simulink model "l1_lbw1_ver100"  (Simulink 7.9)
settings: Solver=FixedStepDiscrete  SolverMode=SingleTasking  StartTime=0.0  StopTime=16484  RelTol=1e-3
undefined symbols (not defined in the file): sfp
libraries: xbsIndex_r4 x1286, casper_library_downconverter x92, dspsigops x32, xps_library x22, casper_library_misc x18, casper_library_flow_control x4
(part 1 of 10)
settings Model: Creator=jayanth  LastModifiedBy=mwagner
settings DebuggingCC: FcnCallInpInsideContextMsg=Use local settings
settings GRTTargetCC: CombineOutputUpdateFcns=off  GRTInterface=on

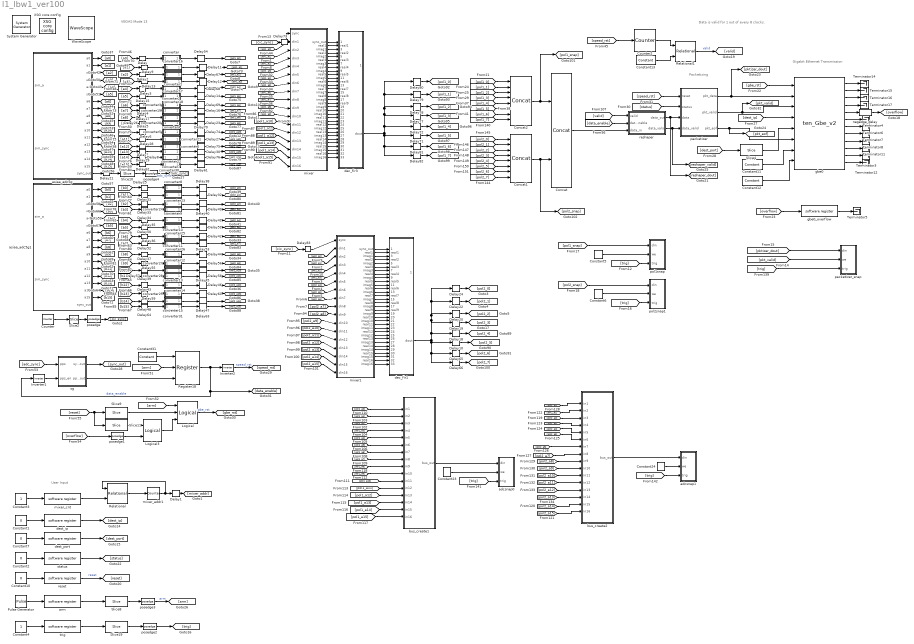
== system l1_lbw1_ver100 ==
  note: Gigabit Ethernet Transmission
  note: Packetizing
  note: Data is valid for 1 out of every 8 clocks.
  note: VEGAS Mode 13
  note: User Input
  " System Generator" : xbsIndex_r4/ System Generator  Tag=genX  xilinxfamily=virtex6  part=xc6vsx475t  speed=-1  package=ff1759  synthesis_tool=XST  clock_wrapper=Clock Enables  directory=./v13_16r128dr_ver110/sysgen  proj_type=Project Navigator  Synth_file=XST Defaults  Impl_file=ISE Defaults  testbench=off  simulink_period=1  sysclk_period=6.6667  dcm_input_clock_period=100  incr_netlist=off  trim_vbits=Everywhere in SubSystem  dbl_ovrd=According to Block Masks  core_generation=According to Block Masks  run_coregen=off  deprecated_control=off  eval_field=0  block_type=sysgen
  Concat : xbsIndex_r4/Concat  num_inputs=2  dbl_ovrd=off  block_type=concat
  Concat1 : xbsIndex_r4/Concat  num_inputs=8  dbl_ovrd=off  block_type=concat
  Concat2 : xbsIndex_r4/Concat  num_inputs=8  dbl_ovrd=off  block_type=concat
  Constant{1..2,7,10} (4 alike) : Constant  Value=0
  Constant11 : xbsIndex_r4/Constant  const=1  gui_display_data_type=Boolean  arith_type=Boolean  n_bits=16  bin_pt=14  preci_type=Single  exp_width=8  frac_width=24  explicit_period=on  period=1  equ=P=C  opselect=C  inp2=PCIN>>17  opr=+  inp1=P  carry=CIN  dbl_ovrd=off  block_type=constant
  Constant12 : xbsIndex_r4/Constant  const=0  gui_display_data_type=Boolean  arith_type=Boolean  n_bits=16  bin_pt=14  preci_type=Single  exp_width=8  frac_width=24  explicit_period=on  period=1  equ=P=C  opselect=C  inp2=PCIN>>17  opr=+  inp1=P  carry=CIN  dbl_ovrd=off  block_type=constant
  Constant13 : xbsIndex_r4/Constant  const=7  gui_display_data_type=Fixed-point  arith_type=Unsigned  n_bits=3  bin_pt=0  preci_type=Single  exp_width=8  frac_width=24  explicit_period=on  period=1  equ=P=C  opselect=C  inp2=PCIN>>17  opr=+  inp1=P  carry=CIN  dbl_ovrd=off  block_type=constant
  Constant{5..6,23..24} (4 alike) : xbsIndex_r4/Constant  const=1  gui_display_data_type=Boolean  arith_type=Boolean  n_bits=32  bin_pt=0  preci_type=Single  exp_width=8  frac_width=24  explicit_period=on  period=1  equ=P=C  opselect=C  inp2=PCIN>>17  opr=+  inp1=P  carry=CIN  dbl_ovrd=off  block_type=constant
      settings: block_version=11.4
  Constant3 : Constant
  Constant31 : xbsIndex_r4/Constant  const=1  gui_display_data_type=Fixed-point  arith_type=Boolean  n_bits=16  bin_pt=0  preci_type=Single  exp_width=8  frac_width=24  explicit_period=on  period=1  equ=P=C  opselect=C  inp2=PCIN>>17  opr=+  inp1=P  carry=CIN  dbl_ovrd=off  block_type=constant
      settings: block_version=11.4
  Constant4 : Constant
  Counter : xbsIndex_r4/Counter  cnt_type=Free Running  cnt_to=Inf  operation=Up  start_count=0  cnt_by_val=1  arith_type=Unsigned  n_bits=16  bin_pt=0  load_pin=off  rst=off  en=off  explicit_period=on  period=1  dbl_ovrd=off  use_behavioral_HDL=off  implementation=Fabric  block_type=counter
  Counter2 : xbsIndex_r4/Counter  cnt_type=Free Running  cnt_to=Inf  operation=Up  start_count=5  cnt_by_val=1  arith_type=Unsigned  n_bits=3  bin_pt=0  load_pin=off  rst=on  en=off  explicit_period=on  period=1  dbl_ovrd=off  use_behavioral_HDL=off  implementation=Fabric  block_type=counter
      settings: block_version=11.4
  Delay{,2..9,13,15,17,21,25..26,28..29,31,33..37,39,43,48,50,52,55,57,59,62,64} (33 alike) : xbsIndex_r4/Delay  rst=off  infoeditControl=Selection of Reset will increase slice count due to use of real FFs and instead of SRLs  en=off  latency=3  dbl_ovrd=off  reg_retiming=off  block_type=delay
  Delay1 : xbsIndex_r4/Delay  rst=off  infoeditControl=Selection of Reset will increase slice count due to use of real FFs and instead of SRLs  en=off  latency=2  dbl_ovrd=off  reg_retiming=on  block_type=delay
      settings: block_version=11.4
  Delay10 : xbsIndex_r4/Delay  rst=off  infoeditControl=Selection of Reset will increase slice count due to use of real FFs and instead of SRLs  en=off  latency=6  dbl_ovrd=off  reg_retiming=on  block_type=delay
      settings: block_version=11.4
  Delay{11..12,14,16,20,23,27,30,32,38,40..42,44..47,49,51,53..54,56,58,60..61,63,67..70,74..76,78} (34 alike) : xbsIndex_r4/Delay  rst=off  infoeditControl=Selection of Reset will increase slice count due to use of real FFs and instead of SRLs  en=off  latency=3  dbl_ovrd=off  reg_retiming=on  block_type=delay
      settings: block_version=11.4
  Delay{18,72..73,83} (4 alike) : xbsIndex_r4/Delay  rst=off  infoeditControl=Selection of Reset will increase slice count due to use of real FFs and instead of SRLs  en=off  latency=5  dbl_ovrd=off  reg_retiming=on  block_type=delay
      settings: block_version=11.4
  Delay19 : xbsIndex_r4/Delay  rst=off  infoeditControl=Selection of Reset will increase slice count due to use of real FFs and instead of SRLs  en=off  latency=4  dbl_ovrd=off  reg_retiming=on  block_type=delay
      settings: block_version=11.4
  Delay22 : xbsIndex_r4/Delay  rst=off  infoeditControl=Selection of Reset will increase slice count due to use of real FFs and instead of SRLs  en=off  latency=2  dbl_ovrd=off  reg_retiming=on  block_type=delay
      settings: block_version=11.4
  Delay24 : xbsIndex_r4/Delay  rst=off  infoeditControl=Selection of Reset will increase slice count due to use of real FFs and instead of SRLs  en=off  latency=1  dbl_ovrd=off  reg_retiming=on  block_type=delay
      settings: block_version=11.4
  Delay65 : xbsIndex_r4/Delay  rst=off  infoeditControl=Selection of Reset will increase slice count due to use of real FFs and instead of SRLs  en=off  latency=7  dbl_ovrd=off  reg_retiming=on  block_type=delay
      settings: block_version=11.4
  Delay66 : xbsIndex_r4/Delay  rst=off  infoeditControl=Selection of Reset will increase slice count due to use of real FFs and instead of SRLs  en=off  latency=8  dbl_ovrd=off  reg_retiming=on  block_type=delay
      settings: block_version=11.4
  Delay71 : xbsIndex_r4/Delay  rst=off  infoeditControl=Selection of Reset will increase slice count due to use of real FFs and instead of SRLs  en=off  latency=6  dbl_ovrd=off  reg_retiming=on  block_type=delay
      settings: block_version=11.4
  Delay77 : xbsIndex_r4/Delay  rst=off  infoeditControl=Selection of Reset will increase slice count due to use of real FFs and instead of SRLs  en=off  latency=4  dbl_ovrd=off  reg_retiming=on  block_type=delay
      settings: block_version=11.4
  Delay79 : xbsIndex_r4/Delay  rst=off  infoeditControl=Selection of Reset will increase slice count due to use of real FFs and instead of SRLs  en=off  latency=2  dbl_ovrd=off  reg_retiming=on  block_type=delay
      settings: block_version=11.4
  Delay80 : xbsIndex_r4/Delay  rst=off  infoeditControl=Selection of Reset will increase slice count due to use of real FFs and instead of SRLs  en=off  latency=1  dbl_ovrd=off  reg_retiming=on  block_type=delay
      settings: block_version=11.4
  Delay81 : xbsIndex_r4/Delay  rst=off  infoeditControl=Selection of Reset will increase slice count due to use of real FFs and instead of SRLs  en=off  latency=7  dbl_ovrd=off  reg_retiming=on  block_type=delay
      settings: block_version=11.4
  Delay82 : xbsIndex_r4/Delay  rst=off  infoeditControl=Selection of Reset will increase slice count due to use of real FFs and instead of SRLs  en=off  latency=8  dbl_ovrd=off  reg_retiming=on  block_type=delay
      settings: block_version=11.4
  Inverter1 : xbsIndex_r4/Inverter  en=off  latency=0  dbl_ovrd=off  block_type=inv
      settings: block_version=11.4
  Inverter2 : xbsIndex_r4/Inverter  en=off  latency=0  dbl_ovrd=off  block_type=inv
      settings: block_version=11.4
  Logical : xbsIndex_r4/Logical  logical_function=OR  inputs=3  en=off  latency=0  precision=Full  arith_type=Unsigned  n_bits=16  bin_pt=0  align_bp=on  dbl_ovrd=off  block_type=logical
  Logical3 : xbsIndex_r4/Logical  logical_function=AND  inputs=2  en=off  latency=0  precision=Full  arith_type=Unsigned  n_bits=8  bin_pt=2  align_bp=on  dbl_ovrd=off  block_type=logical
      settings: xl_area=[0, 0, 0, 0, 0, 0, 0]
  Pulse Generator : DiscretePulseGenerator  Period=10000  PhaseDelay=100
  Register18 : xbsIndex_r4/Register  init=0  rst=on  en=on  dbl_ovrd=off  block_type=register
      settings: block_version=11.4
  Relational : xbsIndex_r4/Relational  mode=a=b  en=off  latency=1  dbl_ovrd=off  block_type=relational
  Relational1 : xbsIndex_r4/Relational  mode=a=b  en=off  latency=0  dbl_ovrd=off  block_type=relational
  Slice{8..10,19} (4 alike) : xbsIndex_r4/Slice  nbits=1  boolean_output=on  mode=Lower Bit Location + Width  bit1=0  base1=MSB of Input  bit0=0  base0=LSB of Input  dbl_ovrd=off  block_type=slice
  Slice11 : xbsIndex_r4/Slice  nbits=1  boolean_output=on  mode=Lower Bit Location + Width  bit1=0  base1=MSB of Input  bit0=1  base0=LSB of Input  dbl_ovrd=off  block_type=slice
      settings: block_version=10.1.3
  Slice2 : xbsIndex_r4/Slice  nbits=1  boolean_output=on  mode=Upper Bit Location + Width  bit1=0  base1=MSB of Input  bit0=0  base0=LSB of Input  dbl_ovrd=off  block_type=slice
  Slice4 : xbsIndex_r4/Slice  nbits=16  boolean_output=off  mode=Lower Bit Location + Width  bit1=0  base1=MSB of Input  bit0=0  base0=LSB of Input  dbl_ovrd=off  block_type=slice
  Terminator{3..8,11..12,14..17} (12 alike) : Terminator
  WaveScope : xbsIndex_r4/WaveScope  block_type=wavescope
  XSG core config : xps_library/XSG core config  Tag=xps:xsg  hw_sys=ROACH2:sx475t  clk_src=adc0_clk  ROACH_clk_src=adc0_clk  ROACH2_clk_src=adc0_clk  clk_rate=150  sample_period=1  synthesis_tool=XST
  adcsnap0 : Subsystem  AncestorBlock=casper_library_scopes/snapshot  mask(snapshot){storage=bram, dram_dimm=1, dram_clock=200, nsamples=12, data_width=128, offset=off, circap=off, value=off, use_dsp48=on}
      mask prompts: storage "Storage medium"; dram_dimm "DRAM dimm"; dram_clock "DRAM clock rate"; nsamples "Number of Samples (2^?)"; data_width "Data width"; offset "Start delay support"; circap "Circular capture support"; value "Extra value capture support"; use_dsp48 "Use DSP48s to implement counters"
      mask help:
      | Standard snap block, but with the following optional extras;
      |  1) Optionally delay the fabric trigger by a user-specified number of valids.
      |  2) Capture continuously after a trigger until a stop pulse is received. Data is captured into BRAM continuously, with old data being overwritten until a stop command is received. Then stop capturing when memory is filled. This enables you to get some data before and some data after the stop pulse. Use the 'tr_en_cnt' register to determine where you are in your vector. 'Addr' register's MSb now indicates 'busy capturing'.
      |  3) Optionally capture a value on an input port to a register at the same time as the first data sample.
      |  4) Implement counters using DSP48Es to save resources.
      mask init:
      | snapshot_init(gcb, ...
      |     'storage', storage, ...
      |     'dram_dimm', dram_dimm, ...
      |     'dram_clock', dram_clock, ...
      |     'nsamples', nsamples, ...
      |     'data_width', data_width, ...
      |     'offset', offset, ...
      |     'circap', circap, ...
      |     'value', value, ...
      |     'use_dsp48', use_dsp48);
      mask StyleString: popup(bram|dram),popup(1|2|3|4),popup(200|250|266|300|333),edit,popup(8|16|32|64|128),checkbox,checkbox,checkbox,checkbox
      mask CallbackString: snapshot_callback();||||||||
  adcsnap1 : Subsystem  AncestorBlock=casper_library_scopes/snapshot  mask(snapshot){storage=bram, dram_dimm=1, dram_clock=200, nsamples=12, data_width=128, offset=off, circap=off, value=off, use_dsp48=on}
      mask prompts: storage "Storage medium"; dram_dimm "DRAM dimm"; dram_clock "DRAM clock rate"; nsamples "Number of Samples (2^?)"; data_width "Data width"; offset "Start delay support"; circap "Circular capture support"; value "Extra value capture support"; use_dsp48 "Use DSP48s to implement counters"
      mask help:
      | Standard snap block, but with the following optional extras;
      |  1) Optionally delay the fabric trigger by a user-specified number of valids.
      |  2) Capture continuously after a trigger until a stop pulse is received. Data is captured into BRAM continuously, with old data being overwritten until a stop command is received. Then stop capturing when memory is filled. This enables you to get some data before and some data after the stop pulse. Use the 'tr_en_cnt' register to determine where you are in your vector. 'Addr' register's MSb now indicates 'busy capturing'.
      |  3) Optionally capture a value on an input port to a register at the same time as the first data sample.
      |  4) Implement counters using DSP48Es to save resources.
      mask init: same as l1_lbw1_ver100/adcsnap0
      mask StyleString: popup(bram|dram),popup(1|2|3|4),popup(200|250|266|300|333),edit,popup(8|16|32|64|128),checkbox,checkbox,checkbox,checkbox
      mask CallbackString: snapshot_callback();||||||||
  arm : xps_library/software register  Tag=xps:sw_reg  io_dir=From Processor  arith_type=Unsigned  bitwidth=32  bin_pt=0  sample_period=1  gw_name=h16k_hbw_ver100_arm_user_data_out
      link override convert: arith_type=Unsigned  n_bits=32  bin_pt=0
      link override newmode13_arm_user_data_out: arith_type=Unsigned  n_bits=32  bin_pt=0  period=1
      link override r_spec_2048_r102_cnt_rst_user_data_out: arith_type=Unsigned  n_bits=32  bin_pt=0  period=1
      link override r_spec_2048_r102_nosim_cnt_rst_user_data_out: arith_type=Unsigned  n_bits=32  bin_pt=0  period=1
      link override r_spec_2048_r103_cnt_rst_user_data_out: arith_type=Unsigned  n_bits=32  bin_pt=0  period=1
      link override roach_spec_no10gbe_sync_cnt_rst_user_data_out: arith_type=Unsigned  n_bits=32  bin_pt=0  period=1
      link override roach_spec_rst_cnt_user_data_out: arith_type=Unsigned  n_bits=32  bin_pt=0  period=1
      link override roach_spec_rst_sync_cnt_user_data_out: arith_type=Unsigned  n_bits=32  bin_pt=0  period=1
  asiaa_adc5g : Subsystem  Tag=xps:adc5g  AncestorBlock=xps_library/ADCs/asiaa_adc5g  mask(adc5g){input_mode=One-channel -- A, adc_brd=ZDOK 0, demux=1:1, adc_bit_width=8, adc_clk_rate=800, using_ctrl=on, test_ramp=off}
      mask prompts: input_mode "Input mode:"; adc_brd "ADC Board"; demux "Internal demux"; adc_bit_width "ADC Resolution (bits):"; adc_clk_rate "ADC Clock Rate (MHz):"; using_ctrl "use control"; test_ramp "start in test ramp mode"
      mask help:
      | Interface for the ASIAA 5 GSps ADC. Supports interleaving all four
      | cores using either input A or C, or interleaving two-cores each for
      | A and C. The hardware itself comes in two versions:
      |
      | DMUX 1:2 -- 4-bit samples, 4 parallel streams
      | DMUX 1:1 -- 8-bit samples, 2 parallel streams
      |
      | In either configuration this block will output 8 parallel streams
      | but the underlying interface, and the bitwidth of the samples,
      | will be different.
      mask init:
      | adc5g_init(gcb,...
      |     'input_mode', input_mode,...
      |     'demux', demux,...
      |     'adc_clk_rate', adc_clk_rate,...
      |     'adc_bit_width', adc_bit_width,...
      |     'adc_brd', adc_brd,...
      |     'using_ctrl', using_ctrl,...
      |     'test_ramp', test_ramp);
      mask StyleString: popup(One-channel -- A|One-channel -- C|Two-channel -- A&C),popup(ZDOK 0|ZDOK 1),popup(1:1|1:2),edit,edit,checkbox,checkbox
      mask CallbackString:
      | ||demux = get_param(gcb,'demux');
      | if(strcmp(demux,'1:1')),
      |     set_param(gcb, 'adc_bit_width', '8')
      | elseif(strcmp(demux, '1:2')),
      |     set_param(gcb, 'adc_bit_width', '4');
      | else
      | end||||
  asiaa_adc5g1 : Subsystem  Tag=xps:adc5g  AncestorBlock=xps_library/ADCs/asiaa_adc5g  mask(adc5g){input_mode=One-channel -- A, adc_brd=ZDOK 1, demux=1:1, adc_bit_width=8, adc_clk_rate=800, using_ctrl=on, test_ramp=off}
      mask prompts: input_mode "Input mode:"; adc_brd "ADC Board"; demux "Internal demux"; adc_bit_width "ADC Resolution (bits):"; adc_clk_rate "ADC Clock Rate (MHz):"; using_ctrl "use control"; test_ramp "start in test ramp mode"
      mask help:
      | Interface for the ASIAA 5 GSps ADC. Supports interleaving all four
      | cores using either input A or C, or interleaving two-cores each for
      | A and C. The hardware itself comes in two versions:
      |
      | DMUX 1:2 -- 4-bit samples, 4 parallel streams
      | DMUX 1:1 -- 8-bit samples, 2 parallel streams
      |
      | In either configuration this block will output 8 parallel streams
      | but the underlying interface, and the bitwidth of the samples,
      | will be different.
      mask init: same as l1_lbw1_ver100/asiaa_adc5g
      mask StyleString: popup(One-channel -- A|One-channel -- C|Two-channel -- A&C),popup(ZDOK 0|ZDOK 1),popup(1:1|1:2),edit,edit,checkbox,checkbox
      mask CallbackString:
      | ||demux = get_param(gcb,'demux');
      | if(strcmp(demux,'1:1')),
      |     set_param(gcb, 'adc_bit_width', '8')
      | elseif(strcmp(demux, '1:2')),
      |     set_param(gcb, 'adc_bit_width', '4');
      | else
      | end||||
  bus_create1 : Subsystem  AncestorBlock=casper_library_flow_control/bus_create  mask(bus_create){inputNum=16}
      mask prompts: inputNum "Number of inputs:"
      mask init:
      | bus_create_init(gcb,...
      |     'inputNum', inputNum);
  bus_create2 : Subsystem  AncestorBlock=casper_library_flow_control/bus_create  mask(bus_create){inputNum=16}
      mask prompts: inputNum "Number of inputs:"
      mask init:
      | bus_create_init(gcb,...
      |     'inputNum', inputNum);
  converter : Subsystem
  converter1 : Subsystem
  converter10 : Subsystem
  converter11 : Subsystem
  converter12 : Subsystem
  converter13 : Subsystem
  converter14 : Subsystem
  converter15 : Subsystem
  converter16 : Subsystem
  converter17 : Subsystem
  converter18 : Subsystem
  converter19 : Subsystem
  converter2 : Subsystem
  converter20 : Subsystem
  converter21 : Subsystem
  converter22 : Subsystem
  converter23 : Subsystem
  converter24 : Subsystem
  converter25 : Subsystem
  converter26 : Subsystem
  converter27 : Subsystem
  converter28 : Subsystem
  converter29 : Subsystem
  converter3 : Subsystem
  converter30 : Subsystem
  converter31 : Subsystem
  converter4 : Subsystem
  converter5 : Subsystem
  converter6 : Subsystem
  converter7 : Subsystem
  converter8 : Subsystem
  converter9 : Subsystem
  dec_fir1 : Subsystem  AncestorBlock=casper_library_downconverter/dec_fir  mask(dec_fir){n_inputs=16, coeff=getfield( getfield( get_param( gcb,'UserData' ), 'parameters'),'coeff'), n_bits=8, quantization=Round  (unbiased: +/- Inf), add_latency=1, mult_latency=2, conv_latency=2, coeff_bit_width=25, coeff_bin_pt=24, absorb_adders=on, adder_imp=DSP48}
      mask prompts: n_inputs "Number of Parallel Streams"; coeff "Coefficients"; n_bits "Bit Width Out"; quantization "Quantization Behavior"; add_latency "Add Latency"; mult_latency "Mult Latency"; conv_latency "Convert latency"; coeff_bit_width "Coefficient bit width"; coeff_bin_pt "Coefficient binary point"; absorb_adders "Absorb adders into DSP slices"; adder_imp "Adder implementation"
      mask help: FIR filter which can handle multiple time samples in parallel and decimates down to 1 time sample. If coefficients are symmetric, will automatically fold before multiplying.
      mask init:
      | dec_fir_init(gcb, ...
      |     'n_inputs', n_inputs, ...
      |     'coeff', coeff, ...
      |     'n_bits', n_bits, ...
      |     'quantization', quantization, ...
      |     'add_latency', add_latency, ...
      |     'mult_latency', mult_latency, ...
      |     'conv_latency', conv_latency, ...
      |     'coeff_bit_width', coeff_bit_width, ...
      |     'coeff_bin_pt', coeff_bin_pt, ...
      |     'absorb_adders', absorb_adders, ...
      |     'adder_imp', adder_imp);
      settings: AttributesFormatString=|
      | 16 taps
      | 8_7 r/i
      mask Help: eval('xlWeb(''http://casper.berkeley.edu/wiki/Dec_fir'')')
      mask StyleString: edit,edit,edit,popup(Truncate|Round  (unbiased: +/- Inf)|Round  (unbiased: Even Values)),edit,edit,edit,edit,edit,checkbox,popup(Behavioral|Fabric|DSP48)
  dec_fir3 : Subsystem  AncestorBlock=casper_library_downconverter/dec_fir  mask(dec_fir){n_inputs=16, coeff=getfield( getfield( get_param( gcb,'UserData' ), 'parameters'),'coeff'), n_bits=8, quantization=Round  (unbiased: +/- Inf), add_latency=1, mult_latency=2, conv_latency=2, coeff_bit_width=25, coeff_bin_pt=24, absorb_adders=on, adder_imp=DSP48}
      mask prompts: n_inputs "Number of Parallel Streams"; coeff "Coefficients"; n_bits "Bit Width Out"; quantization "Quantization Behavior"; add_latency "Add Latency"; mult_latency "Mult Latency"; conv_latency "Convert latency"; coeff_bit_width "Coefficient bit width"; coeff_bin_pt "Coefficient binary point"; absorb_adders "Absorb adders into DSP slices"; adder_imp "Adder implementation"
      mask help: FIR filter which can handle multiple time samples in parallel and decimates down to 1 time sample. If coefficients are symmetric, will automatically fold before multiplying.
      mask init: same as l1_lbw1_ver100/dec_fir1
      settings: AttributesFormatString=|
      | 16 taps
      | 8_7 r/i
      mask Help: eval('xlWeb(''http://casper.berkeley.edu/wiki/Dec_fir'')')
      mask StyleString: edit,edit,edit,popup(Truncate|Round  (unbiased: +/- Inf)|Round  (unbiased: Even Values)),edit,edit,edit,edit,edit,checkbox,popup(Behavioral|Fabric|DSP48)
  dest_ip : xps_library/software register  Tag=xps:sw_reg  io_dir=From Processor  arith_type=Unsigned  bitwidth=32  bin_pt=0  sample_period=1  gw_name=h16k_hbw_ver100_dest_ip_user_data_out
      link override newmode13_dest_ip_user_data_out: arith_type=Unsigned  n_bits=32  bin_pt=0  period=1
      link override packetizer_dest_ip_user_data_out: arith_type=Unsigned  n_bits=32  bin_pt=0  period=1
  dest_port : xps_library/software register  Tag=xps:sw_reg  io_dir=From Processor  arith_type=Unsigned  bitwidth=32  bin_pt=0  sample_period=1  gw_name=h16k_hbw_ver100_dest_port_user_data_out
      link override newmode13_dest_port_user_data_out: arith_type=Unsigned  n_bits=32  bin_pt=0  period=1
      link override packetizer_dest_port_user_data_out: arith_type=Unsigned  n_bits=32  bin_pt=0  period=1
  gbe0 : xps_library/ten_Gbe_v2  Tag=xps:tengbe_v2  flavour=sfp+  slot=1  port_r1=0  port_r2_cx4=0  port_r2_sfpp=0  rx_dist_ram=off  large_frames=on  show_param=on  pre_emph_r2=0.74  pre_emph=3  post_emph_r2=0.18  rxeqmix_r2=7  swing_r2=940  swing=800  fab_en=on  fab_mac=hex2dec('123456780000')  fab_ip=192*(2^24) + 168*(2^16) + 5*(2^8) + 20*(2^0)  fab_udp=10000  fab_gate=1  cpu_rx_en=on  cpu_tx_en=on
  gbe0_overflow : xps_library/software register  Tag=xps:sw_reg  io_dir=To Processor  arith_type=Unsigned  bitwidth=32  bin_pt=0  sample_period=1  gw_name=h16k_hbw_ver100_gbe0_overflow_user_data_in
      link override convert: arith_type=Unsigned  n_bits=32  bin_pt=0
  mixer : Subsystem  AncestorBlock=casper_library_downconverter/mixer  mask(mixer){freq_div=2, freq=2, nstreams=16, n_bits=4, bram_latency=2, mult_latency=4}
      mask prompts: freq_div "Frequency Divisions (M)"; freq "Mixing Frequency (? / M*2pi)"; nstreams "Number of Parallel Streams"; n_bits "Bit Width"; bram_latency "BRAM Latency"; mult_latency "Mult Latency"
      mask help: Digitally mixes an input signal (which can be several samples in parallel) with an LO of the indicated frequency (which is some fraction of the native FPGA clock rate).
      mask init:
      | mixer_init(gcb, ...
      |     'freq_div', freq_div, ...
      |     'freq', freq, ...
      |     'nstreams', nstreams, ...
      |     'n_bits', n_bits, ...
      |     'bram_latency', bram_latency, ...
      |     'mult_latency', mult_latency);
      settings: AttributesFormatString=lo at -2/2
      mask Help: eval('xlWeb(''http://casper.berkeley.edu/wiki/Mixer'')')
  mixer1 : Subsystem  AncestorBlock=casper_library_downconverter/mixer  mask(mixer){freq_div=2, freq=2, nstreams=16, n_bits=4, bram_latency=2, mult_latency=4}
      mask prompts: freq_div "Frequency Divisions (M)"; freq "Mixing Frequency (? / M*2pi)"; nstreams "Number of Parallel Streams"; n_bits "Bit Width"; bram_latency "BRAM Latency"; mult_latency "Mult Latency"
      mask help: Digitally mixes an input signal (which can be several samples in parallel) with an LO of the indicated frequency (which is some fraction of the native FPGA clock rate).
      mask init: same as l1_lbw1_ver100/mixer
      settings: AttributesFormatString=lo at -2/2
      mask Help: eval('xlWeb(''http://casper.berkeley.edu/wiki/Mixer'')')
  mixer_addr1 : xbsIndex_r4/Counter  cnt_type=Free Running  cnt_to=Inf  operation=Up  start_count=0  cnt_by_val=1  arith_type=Unsigned  n_bits=11  bin_pt=0  load_pin=off  rst=on  en=off  explicit_period=on  period=1  dbl_ovrd=off  use_behavioral_HDL=off  implementation=Fabric  block_type=counter
      settings: block_version=11.4
  mixer_cnt : xps_library/software register  Tag=xps:sw_reg  io_dir=From Processor  arith_type=Unsigned  bitwidth=32  bin_pt=0  sample_period=1  gw_name=h16k_hbw_ver100_mixer_cnt_user_data_out
      link override newmode13_mixer_cnt_user_data_out: arith_type=Unsigned  n_bits=32  bin_pt=0  period=1
  negedge_delay : casper_library_misc/negedge_delay  pulse_len=2^20
  packetizer : Subsystem  mask{header_words=2, data_words=1024}
      mask prompts: header_words "Number of 64-bit words in header"; data_words "Number of 64-bit words in data"
  packetizer_snap : Subsystem  AncestorBlock=casper_library_scopes/snapshot  mask(snapshot){storage=bram, dram_dimm=1, dram_clock=200, nsamples=12, data_width=64, offset=off, circap=off, value=off, use_dsp48=on}
      mask prompts: storage "Storage medium"; dram_dimm "DRAM dimm"; dram_clock "DRAM clock rate"; nsamples "Number of Samples (2^?)"; data_width "Data width"; offset "Start delay support"; circap "Circular capture support"; value "Extra value capture support"; use_dsp48 "Use DSP48s to implement counters"
      mask help:
      | Standard snap block, but with the following optional extras;
      |  1) Optionally delay the fabric trigger by a user-specified number of valids.
      |  2) Capture continuously after a trigger until a stop pulse is received. Data is captured into BRAM continuously, with old data being overwritten until a stop command is received. Then stop capturing when memory is filled. This enables you to get some data before and some data after the stop pulse. Use the 'tr_en_cnt' register to determine where you are in your vector. 'Addr' register's MSb now indicates 'busy capturing'.
      |  3) Optionally capture a value on an input port to a register at the same time as the first data sample.
      |  4) Implement counters using DSP48Es to save resources.
      mask init: same as l1_lbw1_ver100/adcsnap0
      mask StyleString: popup(bram|dram),popup(1|2|3|4),popup(200|250|266|300|333),edit,popup(8|16|32|64|128),checkbox,checkbox,checkbox,checkbox
      mask CallbackString: snapshot_callback();||||||||
  pol1snap : Subsystem  AncestorBlock=casper_library_scopes/snapshot  mask(snapshot){storage=bram, dram_dimm=1, dram_clock=200, nsamples=12, data_width=128, offset=off, circap=off, value=off, use_dsp48=on}
      mask prompts: storage "Storage medium"; dram_dimm "DRAM dimm"; dram_clock "DRAM clock rate"; nsamples "Number of Samples (2^?)"; data_width "Data width"; offset "Start delay support"; circap "Circular capture support"; value "Extra value capture support"; use_dsp48 "Use DSP48s to implement counters"
      mask help:
      | Standard snap block, but with the following optional extras;
      |  1) Optionally delay the fabric trigger by a user-specified number of valids.
      |  2) Capture continuously after a trigger until a stop pulse is received. Data is captured into BRAM continuously, with old data being overwritten until a stop command is received. Then stop capturing when memory is filled. This enables you to get some data before and some data after the stop pulse. Use the 'tr_en_cnt' register to determine where you are in your vector. 'Addr' register's MSb now indicates 'busy capturing'.
      |  3) Optionally capture a value on an input port to a register at the same time as the first data sample.
      |  4) Implement counters using DSP48Es to save resources.
      mask init: same as l1_lbw1_ver100/adcsnap0
      mask StyleString: popup(bram|dram),popup(1|2|3|4),popup(200|250|266|300|333),edit,popup(8|16|32|64|128),checkbox,checkbox,checkbox,checkbox
      mask CallbackString: snapshot_callback();||||||||
  pol2snap1 : Subsystem  AncestorBlock=casper_library_scopes/snapshot  mask(snapshot){storage=bram, dram_dimm=1, dram_clock=200, nsamples=12, data_width=128, offset=off, circap=off, value=off, use_dsp48=on}
      mask prompts: storage "Storage medium"; dram_dimm "DRAM dimm"; dram_clock "DRAM clock rate"; nsamples "Number of Samples (2^?)"; data_width "Data width"; offset "Start delay support"; circap "Circular capture support"; value "Extra value capture support"; use_dsp48 "Use DSP48s to implement counters"
      mask help:
      | Standard snap block, but with the following optional extras;
      |  1) Optionally delay the fabric trigger by a user-specified number of valids.
      |  2) Capture continuously after a trigger until a stop pulse is received. Data is captured into BRAM continuously, with old data being overwritten until a stop command is received. Then stop capturing when memory is filled. This enables you to get some data before and some data after the stop pulse. Use the 'tr_en_cnt' register to determine where you are in your vector. 'Addr' register's MSb now indicates 'busy capturing'.
      |  3) Optionally capture a value on an input port to a register at the same time as the first data sample.
      |  4) Implement counters using DSP48Es to save resources.
      mask init: same as l1_lbw1_ver100/adcsnap0
      mask StyleString: popup(bram|dram),popup(1|2|3|4),popup(200|250|266|300|333),edit,popup(8|16|32|64|128),checkbox,checkbox,checkbox,checkbox
      mask CallbackString: snapshot_callback();||||||||
  posedge{,1..4} (5 alike) : casper_library_misc/posedge  Tag=Rising Edge Detector
  reset : xps_library/software register  Tag=xps:sw_reg  io_dir=From Processor  arith_type=Unsigned  bitwidth=32  bin_pt=0  sample_period=1  gw_name=h16k_hbw_ver100_reset_user_data_out
      link override newmode13_reset_user_data_out: arith_type=Unsigned  n_bits=32  bin_pt=0  period=1
      link override packetizer_status_user_data_out: arith_type=Unsigned  n_bits=32  bin_pt=0  period=1
  reshaper : Subsystem
  sg : Subsystem
  status : xps_library/software register  Tag=xps:sw_reg  io_dir=From Processor  arith_type=Unsigned  bitwidth=32  bin_pt=0  sample_period=1  gw_name=h16k_hbw_ver100_status_user_data_out
      link override newmode13_status_user_data_out: arith_type=Unsigned  n_bits=32  bin_pt=0  period=1
      link override packetizer_status_user_data_out: arith_type=Unsigned  n_bits=32  bin_pt=0  period=1
  trig : xps_library/software register  Tag=xps:sw_reg  io_dir=From Processor  arith_type=Unsigned  bitwidth=32  bin_pt=0  sample_period=1  gw_name=h16k_hbw_ver100_trig_user_data_out
      link override cic_filter_testing_to_compile_trig_user_data_out: arith_type=Unsigned  n_bits=32  bin_pt=0  period=1
      link override newmode13_trig_user_data_out: arith_type=Unsigned  n_bits=32  bin_pt=0  period=1
  wires:
  mixer_addr1/1 -> Delay1/1, Relational/1
  Delay1/1 -> [mixer_addr]
  Relational/1 -> mixer_addr1/1
  mixer_cnt/1 -> Relational/2
  Constant3/1 -> mixer_cnt/1
  [cic_sync] -> Delay73/1
  Delay54/1 -> [pol1_a0]
  Delay67/1 -> [pol1_a2]
  Delay68/1 -> [pol1_a4]
  Delay69/1 -> [pol1_a6]
  Delay70/1 -> [pol1_a8]
  Delay74/1 -> [pol1_a10]
  Delay75/1 -> [pol1_a12]
  Delay76/1 -> [pol1_a14]
  Delay/1 -> converter/1(u8_0)
  Delay2/1 -> converter1/1(u8_0)
  Delay3/1 -> converter2/1(u8_0)
  Delay4/1 -> converter3/1(u8_0)
  Delay5/1 -> converter4/1(u8_0)
  Delay6/1 -> converter5/1(u8_0)
  Delay7/1 -> converter6/1(u8_0)
  Delay8/1 -> converter7/1(u8_0)
  converter/1(s8_7) -> Delay54/1
  converter1/1(s8_7) -> Delay67/1
  converter2/1(s8_7) -> Delay68/1
  converter3/1(s8_7) -> Delay69/1
  converter4/1(s8_7) -> Delay70/1
  converter5/1(s8_7) -> Delay74/1
  converter6/1(s8_7) -> Delay75/1
  converter7/1(s8_7) -> Delay76/1
  Counter/1 -> Slice2/1
  Slice2/1 -> posedge/1
  posedge/1 -> [cic_sync]
  gbe0_overflow/1 -> Terminator5/1
  Constant1/1 -> dest_ip/1
  Constant7/1 -> dest_port/1
  dest_ip/1 -> [dest_ip]
  dest_port/1 -> [dest_port]
  [dest_ip] -> gbe0/4
  [dest_port] -> Slice4/1
  Constant2/1 -> status/1
  status/1 -> [status]
  packetizer/3(pkt_eof) -> gbe0/6, [pkt_eof]
  [overflow] -> gbe0_overflow/1
  [spead_rst] -> packetizer/1(reset)
  [status] -> packetizer/2(status)
  reset/1 -> [reset]  "reset"
  Slice4/1 -> gbe0/5
  gbe0/6 -> Terminator4/1
  gbe0/7 -> Terminator6/1
  gbe0/8 -> Terminator7/1
  gbe0/9 -> Terminator8/1
  gbe0/10 -> Terminator11/1
  gbe0/11 -> Terminator3/1
  Constant11/1 -> gbe0/7
  gbe0/1 -> Terminator14/1
  gbe0/2 -> Terminator15/1
  gbe0/3 -> Terminator16/1
  gbe0/4 -> Terminator17/1
  gbe0/5 -> negedge_delay/1
  Constant12/1 -> gbe0/8
  gbe0/12 -> Terminator12/1
  [gbe_rst] -> gbe0/1
  negedge_delay/1 -> [overflow]
  Constant13/1 -> Relational1/2
  Counter2/1 -> Relational1/1
  Relational1/1 -> [valid]  "valid"
  Constant10/1 -> reset/1
  Constant31/1 -> Register18/1
  sg/2(pps_out) -> Register18/3
  Register18/1 -> Inverter2/1, Inverter1/1, [data_enable]  "data_enable"
  arm/1 -> Slice8/1
  Pulse Generator/1 -> arm/1
  Inverter1/1 -> sg/2(pps_en)
  posedge1/1 -> Logical3/2
  Slice11/1 -> Logical3/1
  Slice9/1 -> Logical/2
  Logical3/1 -> Logical/3
  [arm] -> Register18/2
  [adc_sync] -> sg/1(pps)
  sg/1(sync_out) -> [sync_out]
  Inverter2/1 -> [spead_rst]  "spead_rst"
  Logical/1 -> [gbe_rst]  "gbe_rst"
  [overflow] -> posedge1/1
  [reset] -> Slice9/1, Slice11/1
  Delay21/1 -> Slice10/1
  Slice10/1 -> posedge4/1
  posedge4/1 -> [adc_sync]  "adc_sync"
  [spead_rst] -> Counter2/1
  Slice8/1 -> posedge3/1
  posedge3/1 -> [arm]  "arm"
  [arm] -> Logical/1
  [valid] -> reshaper/1(valid)
  [data_enable] -> reshaper/2(data_enable)
  reshaper/1(data_out) -> packetizer/3(data), [reshaper_dout]
  reshaper/2(data_valid) -> packetizer/4(data_valid), [reshaper_valid]
  Constant4/1 -> trig/1
  trig/1 -> Slice19/1
  packetizer/1(pkt_data) -> gbe0/2, [pktizer_dout]
  packetizer/2(pkt_valid) -> gbe0/3, [pkt_valid]
  Concat/1 -> reshaper/3(data_in)
  Delay38/1 -> [pol2_a0]
  Delay40/1 -> [pol2_a2]
  Delay41/1 -> [pol2_a4]
  Delay42/1 -> [pol2_a6]
  Delay44/1 -> [pol2_a8]
  Delay45/1 -> [pol2_a10]
  Delay46/1 -> [pol2_a12]
  Delay47/1 -> [pol2_a14]
  Delay25/1 -> converter8/1(u8_0)
  Delay33/1 -> converter9/1(u8_0)
  Delay35/1 -> converter10/1(u8_0)
  Delay36/1 -> converter11/1(u8_0)
  Delay37/1 -> converter12/1(u8_0)
  Delay39/1 -> converter13/1(u8_0)
  Delay43/1 -> converter14/1(u8_0)
  Delay48/1 -> converter15/1(u8_0)
  converter8/1(s8_7) -> Delay38/1
  converter9/1(s8_7) -> Delay40/1
  converter10/1(s8_7) -> Delay41/1
  converter11/1(s8_7) -> Delay42/1
  converter12/1(s8_7) -> Delay44/1
  converter13/1(s8_7) -> Delay45/1
  converter14/1(s8_7) -> Delay46/1
  converter15/1(s8_7) -> Delay47/1
  asiaa_adc5g/2(a1) -> [a1]
  asiaa_adc5g/4(a3) -> [a3]
  asiaa_adc5g/6(a5) -> [a5]
  asiaa_adc5g/8(a7) -> [a7]
  asiaa_adc5g/10(a9) -> [a9]
  asiaa_adc5g/12(a11) -> [a11]
  asiaa_adc5g/14(a13) -> [a13]
  asiaa_adc5g/16(a15) -> [a15]
  asiaa_adc5g/1(a0) -> [a0]
  asiaa_adc5g/15(a14) -> [a14]
  asiaa_adc5g/13(a12) -> [a12]
  asiaa_adc5g/11(a10) -> [a10]
  asiaa_adc5g/7(a6) -> [a6]
  asiaa_adc5g/5(a4) -> [a4]
  asiaa_adc5g/3(a2) -> [a2]
  asiaa_adc5g/9(a8) -> [a8]
  [a0] -> Delay/1
  [a2] -> Delay2/1
  [a4] -> Delay3/1
  [a6] -> Delay4/1
  [a8] -> Delay5/1
  [a10] -> Delay6/1
  [a12] -> Delay7/1
  [a14] -> Delay8/1
  [b0] -> Delay25/1
  [b2] -> Delay33/1
  [b4] -> Delay35/1
  [b6] -> Delay36/1
  [b8] -> Delay37/1
  [b10] -> Delay39/1
  [b12] -> Delay43/1
  [b14] -> Delay48/1
  asiaa_adc5g/17(sync_out) -> Delay21/1
  asiaa_adc5g1/1(a0) -> [b0]
  asiaa_adc5g1/2(a1) -> [b1]
  asiaa_adc5g1/3(a2) -> [b2]
  asiaa_adc5g1/4(a3) -> [b3]
  asiaa_adc5g1/5(a4) -> [b4]
  asiaa_adc5g1/6(a5) -> [b5]
  asiaa_adc5g1/7(a6) -> [b6]
  asiaa_adc5g1/8(a7) -> [b7]
  asiaa_adc5g1/9(a8) -> [b8]
  asiaa_adc5g1/10(a9) -> [b9]
  asiaa_adc5g1/11(a10) -> [b10]
  asiaa_adc5g1/12(a11) -> [b11]
  asiaa_adc5g1/13(a12) -> [b12]
  asiaa_adc5g1/14(a13) -> [b13]
  asiaa_adc5g1/15(a14) -> [b14]
  asiaa_adc5g1/16(a15) -> [b15]
  Delay11/1 -> [pol1_a1]
  Delay9/1 -> converter16/1(u8_0)
  converter16/1(s8_7) -> Delay11/1
  [a1] -> Delay9/1
  Delay12/1 -> [pol1_a3]
  Delay13/1 -> converter17/1(u8_0)
  converter17/1(s8_7) -> Delay12/1
  [a3] -> Delay13/1
  Delay14/1 -> [pol1_a5]
  Delay15/1 -> converter18/1(u8_0)
  converter18/1(s8_7) -> Delay14/1
  [a5] -> Delay15/1
  Delay16/1 -> [pol1_a7]
  Delay17/1 -> converter19/1(u8_0)
  converter19/1(s8_7) -> Delay16/1
  [a7] -> Delay17/1
  Delay23/1 -> [pol1_a9]
  Delay26/1 -> converter20/1(u8_0)
  converter20/1(s8_7) -> Delay23/1
  [a9] -> Delay26/1
  Delay27/1 -> [pol1_a11]
  Delay28/1 -> converter21/1(u8_0)
  converter21/1(s8_7) -> Delay27/1
  [a11] -> Delay28/1
  Delay30/1 -> [pol1_a13]
  Delay29/1 -> converter22/1(u8_0)
  converter22/1(s8_7) -> Delay30/1
  [a13] -> Delay29/1
  Delay32/1 -> [pol2_a1]
  Delay31/1 -> converter23/1(u8_0)
  converter23/1(s8_7) -> Delay32/1
  [b1] -> Delay31/1
  Delay49/1 -> [pol2_a3]
  Delay34/1 -> converter24/1(u8_0)
  converter24/1(s8_7) -> Delay49/1
  [b3] -> Delay34/1
  Delay51/1 -> [pol2_a5]
  Delay50/1 -> converter25/1(u8_0)
  converter25/1(s8_7) -> Delay51/1
  [b5] -> Delay50/1
  Delay53/1 -> [pol2_a7]
  Delay52/1 -> converter26/1(u8_0)
  converter26/1(s8_7) -> Delay53/1
  [b7] -> Delay52/1
  Delay56/1 -> [pol2_a9]
  Delay55/1 -> converter27/1(u8_0)
  converter27/1(s8_7) -> Delay56/1
  [b9] -> Delay55/1
  Delay58/1 -> [pol2_a11]
  Delay57/1 -> converter28/1(u8_0)
  converter28/1(s8_7) -> Delay58/1
  [b11] -> Delay57/1
  Delay60/1 -> [pol2_a13]
  Delay59/1 -> converter29/1(u8_0)
  converter29/1(s8_7) -> Delay60/1
  [b13] -> Delay59/1
  Delay61/1 -> [pol1_a15]
  Delay62/1 -> converter30/1(u8_0)
  converter30/1(s8_7) -> Delay61/1
  [a15] -> Delay62/1
  Delay63/1 -> [pol2_a15]
  Delay64/1 -> converter31/1(u8_0)
  converter31/1(s8_7) -> Delay63/1
  [b15] -> Delay64/1
  Delay73/1 -> mixer/1(sync)
  [pol1_a0] -> mixer/2(din1)
  [pol1_a1] -> mixer/3(din2)
  [pol1_a2] -> mixer/4(din3)
  [pol1_a3] -> mixer/5(din4)
  [pol1_a4] -> mixer/6(din5)
  [pol1_a5] -> mixer/7(din6)
  [pol1_a6] -> mixer/8(din7)
  [pol1_a7] -> mixer/9(din8)
  [pol1_a8] -> mixer/10(din9)
  [pol1_a9] -> mixer/11(din10)
  [pol1_a10] -> mixer/12(din11)
  [pol1_a11] -> mixer/13(din12)
  [pol1_a12] -> mixer/14(din13)
  [pol1_a13] -> mixer/15(din14)
  [pol1_a14] -> mixer/16(din15)
  [pol1_a15] -> mixer/17(din16)
  Constant23/1 -> adcsnap0/2(we)
  bus_create1/1(bus_out) -> adcsnap0/1(din)
  [pol1_a0] -> bus_create1/1(in1)
  [pol1_a1] -> bus_create1/2(in2)
  [pol1_a2] -> bus_create1/3(in3)
  [pol1_a3] -> bus_create1/4(in4)
  [pol1_a4] -> bus_create1/5(in5)
  [pol1_a5] -> bus_create1/6(in6)
  [pol1_a6] -> bus_create1/7(in7)
  [pol1_a7] -> bus_create1/8(in8)
  [pol1_a8] -> bus_create1/9(in9)
  [pol1_a9] -> bus_create1/10(in10)
  [pol1_a10] -> bus_create1/11(in11)
  [pol1_a11] -> bus_create1/12(in12)
  [pol1_a12] -> bus_create1/13(in13)
  [pol1_a13] -> bus_create1/14(in14)
  [pol1_a14] -> bus_create1/15(in15)
  [pol1_a15] -> bus_create1/16(in16)
  Constant24/1 -> adcsnap1/2(we)
  bus_create2/1(bus_out) -> adcsnap1/1(din)
  [pol2_a0] -> bus_create2/1(in1)
  [pol2_a1] -> bus_create2/2(in2)
  [pol2_a2] -> bus_create2/3(in3)
  [pol2_a3] -> bus_create2/4(in4)
  [pol2_a4] -> bus_create2/5(in5)
  [pol2_a5] -> bus_create2/6(in6)
  [pol2_a6] -> bus_create2/7(in7)
  [pol2_a7] -> bus_create2/8(in8)
  [pol2_a8] -> bus_create2/9(in9)
  [pol2_a9] -> bus_create2/10(in10)
  [pol2_a10] -> bus_create2/11(in11)
  [pol2_a11] -> bus_create2/12(in12)
  [pol2_a12] -> bus_create2/13(in13)
  [pol2_a13] -> bus_create2/14(in14)
  [pol2_a14] -> bus_create2/15(in15)
  [pol2_a15] -> bus_create2/16(in16)
  [pkt_valid] -> packetizer_snap/2(we)
  [pktizer_dout] -> packetizer_snap/1(din)
  Slice19/1 -> posedge2/1
  posedge2/1 -> [trig]
  [trig] -> adcsnap0/3(trig)
  [trig] -> adcsnap1/3(trig)
  [trig] -> packetizer_snap/3(trig)
  mixer/1(sync_out) -> dec_fir3/1(sync_in)
  mixer/2(real1) -> dec_fir3/2(real1)
  mixer/3(imag1) -> dec_fir3/3(imag1)
  mixer/4(real2) -> dec_fir3/4(real2)
  mixer/5(imag2) -> dec_fir3/5(imag2)
  mixer/6(real3) -> dec_fir3/6(real3)
  mixer/7(imag3) -> dec_fir3/7(imag3)
  mixer/8(real4) -> dec_fir3/8(real4)
  mixer/9(imag4) -> dec_fir3/9(imag4)
  mixer/10(real5) -> dec_fir3/10(real5)
  mixer/11(imag5) -> dec_fir3/11(imag5)
  mixer/12(real6) -> dec_fir3/12(real6)
  mixer/13(imag6) -> dec_fir3/13(imag6)
  mixer/14(real7) -> dec_fir3/14(real7)
  mixer/15(imag7) -> dec_fir3/15(imag7)
  mixer/16(real8) -> dec_fir3/16(real8)
  mixer/17(imag8) -> dec_fir3/17(imag8)
  mixer/18(real9) -> dec_fir3/18(real9)
  mixer/19(imag9) -> dec_fir3/19(imag9)
  mixer/20(real10) -> dec_fir3/20(real10)
  mixer/21(imag10) -> dec_fir3/21(imag10)
  mixer/22(real11) -> dec_fir3/22(real11)
  mixer/23(imag11) -> dec_fir3/23(imag11)
  mixer/24(real12) -> dec_fir3/24(real12)
  mixer/25(imag12) -> dec_fir3/25(imag12)
  mixer/26(real13) -> dec_fir3/26(real13)
  mixer/27(imag13) -> dec_fir3/27(imag13)
  mixer/28(real14) -> dec_fir3/28(real14)
  mixer/29(imag14) -> dec_fir3/29(imag14)
  mixer/30(real15) -> dec_fir3/30(real15)
  mixer/31(imag15) -> dec_fir3/31(imag15)
  mixer/32(real16) -> dec_fir3/32(real16)
  mixer/33(imag16) -> dec_fir3/33(imag16)
  mixer1/1(sync_out) -> dec_fir1/1(sync_in)
  mixer1/2(real1) -> dec_fir1/2(real1)
  mixer1/3(imag1) -> dec_fir1/3(imag1)
  mixer1/4(real2) -> dec_fir1/4(real2)
  mixer1/5(imag2) -> dec_fir1/5(imag2)
  mixer1/6(real3) -> dec_fir1/6(real3)
  mixer1/7(imag3) -> dec_fir1/7(imag3)
  mixer1/8(real4) -> dec_fir1/8(real4)
  mixer1/9(imag4) -> dec_fir1/9(imag4)
  mixer1/10(real5) -> dec_fir1/10(real5)
  mixer1/11(imag5) -> dec_fir1/11(imag5)
  mixer1/12(real6) -> dec_fir1/12(real6)
  mixer1/13(imag6) -> dec_fir1/13(imag6)
  mixer1/14(real7) -> dec_fir1/14(real7)
  mixer1/15(imag7) -> dec_fir1/15(imag7)
  mixer1/16(real8) -> dec_fir1/16(real8)
  mixer1/17(imag8) -> dec_fir1/17(imag8)
  mixer1/18(real9) -> dec_fir1/18(real9)
  mixer1/19(imag9) -> dec_fir1/19(imag9)
  mixer1/20(real10) -> dec_fir1/20(real10)
  mixer1/21(imag10) -> dec_fir1/21(imag10)
  mixer1/22(real11) -> dec_fir1/22(real11)
  mixer1/23(imag11) -> dec_fir1/23(imag11)
  mixer1/24(real12) -> dec_fir1/24(real12)
  mixer1/25(imag12) -> dec_fir1/25(imag12)
  mixer1/26(real13) -> dec_fir1/26(real13)
  mixer1/27(imag13) -> dec_fir1/27(imag13)
  mixer1/28(real14) -> dec_fir1/28(real14)
  mixer1/29(imag14) -> dec_fir1/29(imag14)
  mixer1/30(real15) -> dec_fir1/30(real15)
  mixer1/31(imag15) -> dec_fir1/31(imag15)
  mixer1/32(real16) -> dec_fir1/32(real16)
  mixer1/33(imag16) -> dec_fir1/33(imag16)
  dec_fir1/2(dout) -> Delay24/1, Delay22/1, Delay20/1, Delay19/1, Delay18/1, Delay10/1, Delay65/1, Delay66/1
  Delay24/1 -> [pol2_0]
  Delay22/1 -> [pol2_1]
  Delay20/1 -> [pol2_2]
  Delay19/1 -> [pol2_3]
  Delay18/1 -> [pol2_4]
  Delay10/1 -> [pol2_5]
  Delay65/1 -> [pol2_6]
  Delay66/1 -> [pol2_7]
  dec_fir3/2(dout) -> Delay82/1, Delay81/1, Delay71/1, Delay72/1, Delay77/1, Delay78/1, Delay79/1, Delay80/1
  Delay80/1 -> [pol1_0]
  Delay79/1 -> [pol1_1]
  Delay78/1 -> [pol1_2]
  Delay77/1 -> [pol1_3]
  Delay72/1 -> [pol1_4]
  Delay71/1 -> [pol1_5]
  Delay81/1 -> [pol1_6]
  Delay82/1 -> [pol1_7]
  [pol1_0] -> Concat2/1
  [pol1_1] -> Concat2/2
  [pol1_2] -> Concat2/3
  [pol1_3] -> Concat2/4
  [pol1_4] -> Concat2/5
  [pol1_5] -> Concat2/6
  [pol1_6] -> Concat2/7
  [pol1_7] -> Concat2/8
  [pol2_0] -> Concat1/1
  [pol2_1] -> Concat1/2
  [pol2_2] -> Concat1/3
  [pol2_3] -> Concat1/4
  [pol2_4] -> Concat1/5
  [pol2_5] -> Concat1/6
  [pol2_6] -> Concat1/7
  [pol2_7] -> Concat1/8
  [cic_sync] -> Delay83/1
  Delay83/1 -> mixer1/1(sync)
  [pol2_a0] -> mixer1/2(din1)
  [pol2_a1] -> mixer1/3(din2)
  [pol2_a2] -> mixer1/4(din3)
  [pol2_a3] -> mixer1/5(din4)
  [pol2_a4] -> mixer1/6(din5)
  [pol2_a5] -> mixer1/7(din6)
  [pol2_a6] -> mixer1/8(din7)
  [pol2_a7] -> mixer1/9(din8)
  [pol2_a8] -> mixer1/10(din9)
  [pol2_a9] -> mixer1/11(din10)
  [pol2_a10] -> mixer1/12(din11)
  [pol2_a11] -> mixer1/13(din12)
  [pol2_a12] -> mixer1/14(din13)
  [pol2_a13] -> mixer1/15(din14)
  [pol2_a14] -> mixer1/16(din15)
  [pol2_a15] -> mixer1/17(din16)
  Concat2/1 -> Concat/1, [pol1_snap]
  Concat1/1 -> Concat/2, [pol2_snap]
  Constant5/1 -> pol1snap/2(we)
  [pol1_snap] -> pol1snap/1(din)
  [trig] -> pol1snap/3(trig)
  Constant6/1 -> pol2snap1/2(we)
  [pol2_snap] -> pol2snap1/1(din)
  [trig] -> pol2snap1/3(trig)
